simulink model "REALTIME_PART1_antiawu"  (R2020b)
settings: Solver=ode3  StartTime=0.0  StopTime=5  FixedStep=0.001  RelTol=1e-3
undefined symbols (not defined in the file or in its folder): ctrl, degs2rpm, denHwa, denHws, National_Instruments, numHwa, numHws, PCI, sens, step_size
libraries: sldrtlib x2
settings Model: ExtModeTrigDuration=6000  Creator=gioel  LastModifiedBy=ambrosingi
settings DataIOCC: ReturnWorkspaceOutputs=off
settings RTWCC: Description=Simulink Desktop Real-Time  SystemTargetFile=sldrt.tlc  TemplateMakefile=sldrt.tmf  RTWCompilerOptimization=on
settings CodeAppCC: MaxIdLength=95
settings SimulinkDesktopRealTimeCC: TargetPreCompLibLocation=C:\Program Files\MATLAB\R2020b\toolbox\sldrt\lib\win64

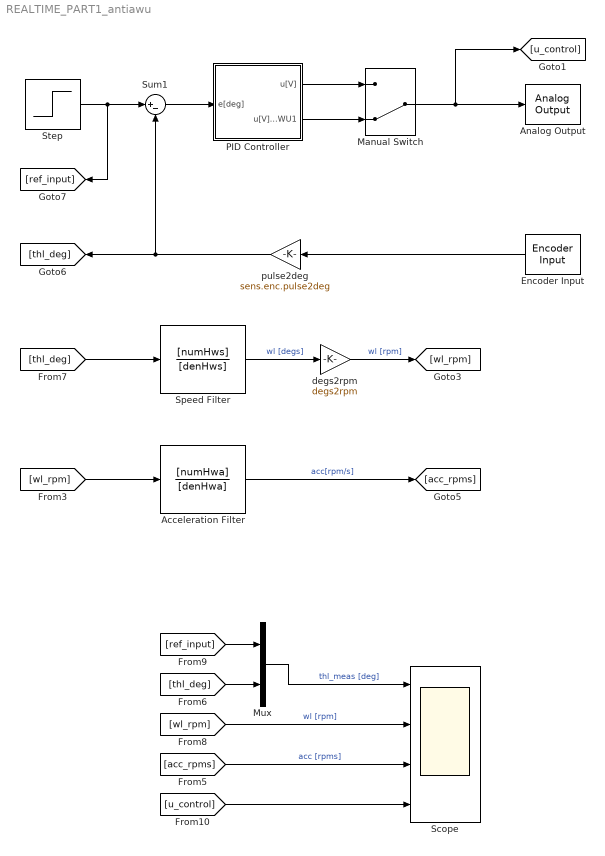
== system REALTIME_PART1_antiawu ==
  Acceleration Filter : TransferFcn  Numerator=[numHwa]  Denominator=[denHwa]
  Analog Output : sldrtlib/Analog Output  SampleTime=0.001  MaxMissedTicks=10  ShowMissedTicks=off  YieldWhenWaiting=off  DrvName=National_Instruments/PCI-6221  DrvAddress=4294967295  DrvOptions=[0 0 0 2 0]  Channels=1  RangeMode=1  VoltRange=1  InitialValue=0  FinalValue=0
      settings: AttributesFormatString=National Instruments\nPCI-6221 [auto]
  Encoder Input : sldrtlib/Encoder Input  SampleTime=0.001  MaxMissedTicks=10  ShowMissedTicks=off  YieldWhenWaiting=off  DrvName=National_Instruments/PCI-6221  DrvAddress=4294967295  DrvOptions=[0 0 0 2 0]  Channels=1  QuadMode=3  IndexPulse=1  InputFilter=Inf  DataType=1
      settings: AttributesFormatString=National Instruments\nPCI-6221 [auto]
  Manual Switch : ManualSwitch  CurrentSetting=0
  Mux : Mux  Inputs=2
  PID Controller : Subsystem
  Scope : Scope  NumInputPorts=4
  Speed Filter : TransferFcn  Numerator=[numHws]  Denominator=[denHws]
  Step : Step  After=step_size  SampleTime=0
  Sum1 : Sum  Inputs=|+-
  degs2rpm : Gain  Gain=degs2rpm
  pulse2deg : Gain  Gain=sens.enc.pulse2deg
  wires:
  Sum1/1 -> PID Controller/1(e[deg])
  Step/1 -> [ref_input], Sum1/1
  Speed Filter/1 -> degs2rpm/1  "wl [degs]"
  Encoder Input/1 -> pulse2deg/1
  pulse2deg/1 -> [thl_deg], Sum1/2
  [thl_deg] -> Speed Filter/1
  degs2rpm/1 -> [wl_rpm]  "wl [rpm]"
  [wl_rpm] -> Acceleration Filter/1
  Acceleration Filter/1 -> [acc_rpms]  "acc[rpm/s]"
  [ref_input] -> Mux/1
  [thl_deg] -> Mux/2
  Mux/1 -> Scope/1  "thl_meas [deg]"
  [acc_rpms] -> Scope/3  "acc [rpms]"
  PID Controller/2(u[V]_AWU1) -> Manual Switch/2
  PID Controller/1(u[V]) -> Manual Switch/1
  Manual Switch/1 -> Analog Output/1, [u_control]
  [u_control] -> Scope/4
  [wl_rpm] -> Scope/2  "wl [rpm]"

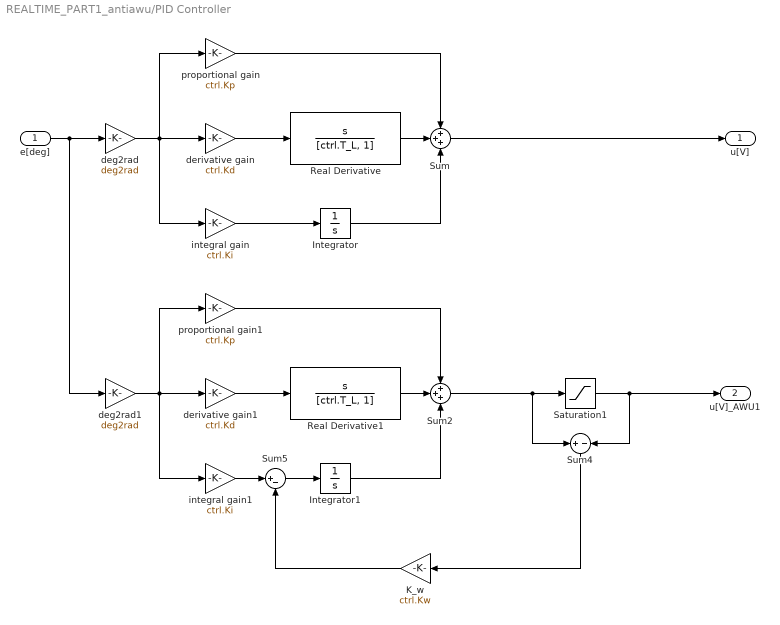
== system REALTIME_PART1_antiawu/PID Controller ==
  e[deg] : Inport
  Integrator : Integrator
  Integrator1 : Integrator
  K_w : Gain  Gain=ctrl.Kw
  Real Derivative : TransferFcn  Numerator=[1 0]  Denominator=[ctrl.T_L, 1]
  Real Derivative1 : TransferFcn  Numerator=[1 0]  Denominator=[ctrl.T_L, 1]
  Saturation1 : Saturate  UpperLimit=10  LowerLimit=-10
  Sum : Sum  Inputs=+++
  Sum2 : Sum  Inputs=+++
  Sum4 : Sum  Inputs=+|-
  Sum5 : Sum  Inputs=|+-
  deg2rad : Gain  Gain=deg2rad
  deg2rad1 : Gain  Gain=deg2rad
  derivative gain : Gain  Gain=ctrl.Kd
  derivative gain1 : Gain  Gain=ctrl.Kd
  integral gain : Gain  Gain=ctrl.Ki
  integral gain1 : Gain  Gain=ctrl.Ki
  proportional gain : Gain  Gain=ctrl.Kp
  proportional gain1 : Gain  Gain=ctrl.Kp
  u[V] : Outport
  u[V]_AWU1 : Outport  Port=2
  wires:
  Real Derivative/1 -> Sum/2
  proportional gain/1 -> Sum/1
  derivative gain/1 -> Real Derivative/1
  deg2rad/1 -> integral gain/1, derivative gain/1, proportional gain/1
  Integrator/1 -> Sum/3
  integral gain/1 -> Integrator/1
  Sum/1 -> u[V]/1
  K_w/1 -> Sum5/2
  Sum2/1 -> Saturation1/1, Sum4/1
  Saturation1/1 -> Sum4/2, u[V]_AWU1/1
  e[deg]/1 -> deg2rad1/1, deg2rad/1
  Sum5/1 -> Integrator1/1
  integral gain1/1 -> Sum5/1
  Integrator1/1 -> Sum2/3
  deg2rad1/1 -> proportional gain1/1, derivative gain1/1, integral gain1/1
  derivative gain1/1 -> Real Derivative1/1
  Sum4/1 -> K_w/1
  proportional gain1/1 -> Sum2/1
  Real Derivative1/1 -> Sum2/2
